simulink library "sandbox_lib"  (R2020b)
settings: Solver=VariableStepAuto  StartTime=0.0  StopTime=10.0  RelTol=1e-3
settings Model: Creator=CHOLSCH3  LastModifiedBy=CHOLSCH3
settings SFSimCC: SimTargetLang=C++
settings SFSimCC: SimCustomSourceCode=|
  | const uint32_t num_entries = 256;
  | static std::uint32_t storage[num_entries][num_entries] = {};
  | 
  | bool write_parameter_float(std::uint32_t group, std::uint32_t index, float value)
  | {
  |     if(group>=num_entries || index >= num_entries)
  |         return false;
  | 
  |     *(float *)&storage[group][index] = value;
  |     return true;
  | }
  | float read_parameter_float(std::uint32_t group, std::uint32_t index)
  | {
  |     if(group>=num_entries || index >= num_entries)
  |         return 0.0f;
  | 
  |     return *(float *)&storage[group][index];
  | }
  | bool write_parameter_int32(uint32_t group, uint32_t index, int32_t value)
  | {
  |     if(group>=num_entries || index >= num_entries)
  |         return false;
  | 
  |     *(int32_t *)&storage[group][index] = value;
  |     return true;
  | }
  | int32_t read_parameter_int32(uint32_t group, uint32_t index)
  | {
  |     if(group>=num_entries || index >= num_entries)
  |         return 0;
  | 
  |     return *(int32_t *)&storage[group][index];
  | }
settings SFSimCC: SimCustomHeaderCode=|
  | #include <cstdint>
  | bool write_parameter_float(std::uint32_t group, std::uint32_t index, float value);
  | float read_parameter_float(std::uint32_t group, std::uint32_t index);
  | bool write_parameter_int32(uint32_t group, uint32_t index, int32_t value);
  | int32_t read_parameter_int32(uint32_t group, uint32_t index);
settings RTWCC: CustomHeaderCode="#include \"syscalls.h\""

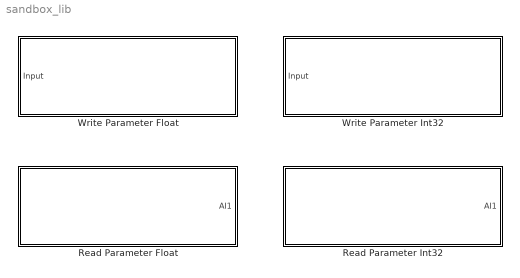
== system sandbox_lib ==
  Read Parameter Float : Subsystem  TreatAsAtomicUnit=on  mask{parameter_group=00, parameter_index=00}
      mask prompts: parameter_group "Parameter Group"; parameter_index "Parameter Index"
      mask Display: disp(['Read Parameter Float\n' get_param(gcb,'parameter_group') '.' get_param(gcb,'parameter_index')])
  Read Parameter Int32 : Subsystem  TreatAsAtomicUnit=on  mask{parameter_group=00, parameter_index=00}
      mask prompts: parameter_group "Parameter Group"; parameter_index "Parameter Index"
      mask Display: disp(['Read Parameter Int32\n' get_param(gcb,'parameter_group') '.' get_param(gcb,'parameter_index')])
  Write Parameter Float : Subsystem  TreatAsAtomicUnit=on  mask{parameter_group=00, parameter_index=00}
      mask prompts: parameter_group "Parameter Group"; parameter_index "Parameter Index"
      mask Display: disp(['Write Parameter Float\n' get_param(gcb,'parameter_group') '.' get_param(gcb,'parameter_index')])
  Write Parameter Int32 : Subsystem  TreatAsAtomicUnit=on  mask{parameter_group=00, parameter_index=00}
      mask prompts: parameter_group "Parameter Group"; parameter_index "Parameter Index"
      mask Display: disp(['Write Parameter Int32\n' get_param(gcb,'parameter_group') '.' get_param(gcb,'parameter_index')])

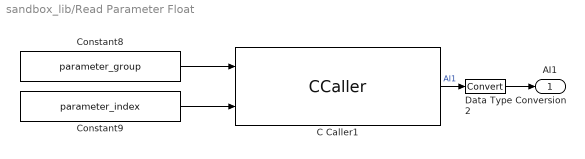
== system sandbox_lib/Read Parameter Float ==
  C Caller1 : CCaller  FunctionName=read_parameter_float  PortSpecificationStruct="%)30     .    > 4   8    (     @         %    \"     ,    !     0         %  0 \"0    $    _    07)G3F%M90  4&]R=$YA;64 4V-O<&4     26YD97@     5'EP90      4VEZ90      27-';&]B86P   X    P    !@    @    $          4    (     0    ,    !         !   P!O=70 #@   #     &    \"     0         !0    @    !     P    $         $  # &]U=  .    .     8    (    !          %    \"     $    &     0         0    !@   $]U='!U=   #@   #@    &    \"     8         !0    @    !     0    $         \"0    @               X    X    !@    @    $          4    (     0    8    !         !     &    <VEN9VQE   .    ,     8    (    !          %    \"     $    !     0         0  $ ,0    X    P    !@    @    ) @        4    (     0    $    !          (  0      #@   #@    &    \"     0         !0    @    !    !0    $         $     4   !G<F]U<     X    X    !@    @    $          4    (     0    4    !         !     %    9W)O=7     .    .     8    (    !          %    \"     $    %     0         0    !0   $EN<'5T    #@   #@    &    \"     8         !0    @    !     0    $         \"0    @               X    X    !@    @    $          4    (     0    8    !         !     &    =6EN=#,R   .    ,     8    (    !          %    \"     $    !     0         0  $ ,0    X    P    !@    @    ) @        4    (     0    $    !          (  0      #@   #@    &    \"     0         !0    @    !    !0    $         $     4   !I;F1E>     X    X    !@    @    $          4    (     0    4    !         !     %    :6YD97@    .    .     8    (    !          %    \"     $    %     0         0    !0   $EN<'5T    #@   #@    &    \"     8         !0    @    !     0    $         \"0    @           #P/PX    X    !@    @    $          4    (     0    8    !         !     &    =6EN=#,R   .    ,     8    (    !          %    \"     $    !     0         0  $ ,0    X    P    !@    @    ) @        4    (     0    $    !          (  0"
  Constant8 : Constant  Value=parameter_group  OutDataTypeStr=Inherit: Inherit via back propagation
  Constant9 : Constant  Value=parameter_index  OutDataTypeStr=Inherit: Inherit via back propagation
  Data Type Conversion2 : DataTypeConversion
  AI1 : Outport
  wires:
  Constant8/1 -> C Caller1/1
  Constant9/1 -> C Caller1/2
  Data Type Conversion2/1 -> AI1/1
  C Caller1/1 -> Data Type Conversion2/1  "AI1"

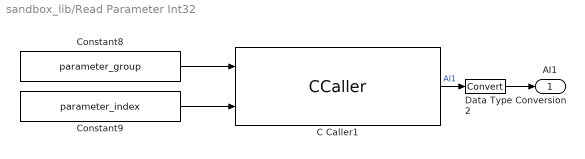
== system sandbox_lib/Read Parameter Int32 ==
  C Caller1 : CCaller  FunctionName=read_parameter_int32
  Constant8 : Constant  Value=parameter_group  OutDataTypeStr=Inherit: Inherit via back propagation
  Constant9 : Constant  Value=parameter_index  OutDataTypeStr=Inherit: Inherit via back propagation
  Data Type Conversion2 : DataTypeConversion
  AI1 : Outport
  wires:
  Constant8/1 -> C Caller1/1
  Constant9/1 -> C Caller1/2
  Data Type Conversion2/1 -> AI1/1
  C Caller1/1 -> Data Type Conversion2/1  "AI1"

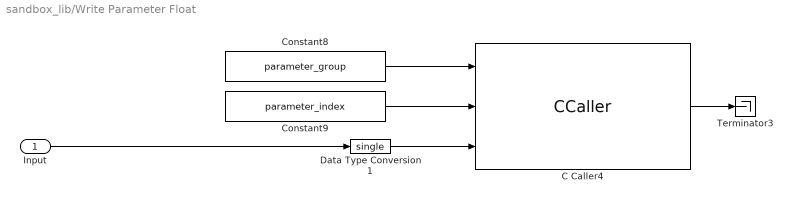
== system sandbox_lib/Write Parameter Float ==
  Input : Inport
  C Caller4 : CCaller  FunctionName=write_parameter_float  PortSpecificationStruct="%)30     .    * <   8    (     @         %    \"     0    !     0         %  0 \"0    $    _    07)G3F%M90  4&]R=$YA;64 4V-O<&4     26YD97@     5'EP90      4VEZ90      27-';&]B86P   X    P    !@    @    $          4    (     0    ,    !         !   P!O=70 #@   #     &    \"     0         !0    @    !     P    $         $  # &]U=  .    .     8    (    !          %    \"     $    &     0         0   ...(+2078 chars)"
  Constant8 : Constant  Value=parameter_group  OutDataTypeStr=Inherit: Inherit via back propagation
  Constant9 : Constant  Value=parameter_index  OutDataTypeStr=Inherit: Inherit via back propagation
  Data Type Conversion1 : DataTypeConversion  OutDataTypeStr=single
  Terminator3 : Terminator
  wires:
  Constant9/1 -> C Caller4/2
  Input/1 -> Data Type Conversion1/1
  C Caller4/1 -> Terminator3/1
  Constant8/1 -> C Caller4/1
  Data Type Conversion1/1 -> C Caller4/3

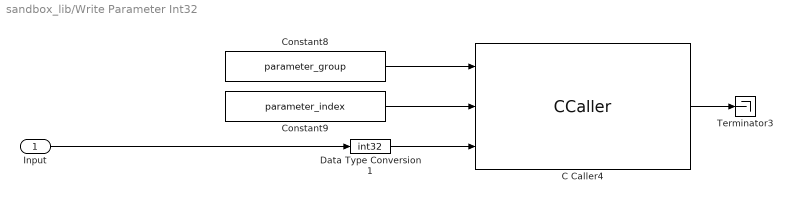
== system sandbox_lib/Write Parameter Int32 ==
  Input : Inport
  C Caller4 : CCaller  FunctionName=write_parameter_int32
  Constant8 : Constant  Value=parameter_group  OutDataTypeStr=Inherit: Inherit via back propagation
  Constant9 : Constant  Value=parameter_index  OutDataTypeStr=Inherit: Inherit via back propagation
  Data Type Conversion1 : DataTypeConversion  OutDataTypeStr=int32  RndMeth=Round
  Terminator3 : Terminator
  wires:
  Constant9/1 -> C Caller4/2
  Input/1 -> Data Type Conversion1/1
  C Caller4/1 -> Terminator3/1
  Constant8/1 -> C Caller4/1
  Data Type Conversion1/1 -> C Caller4/3
